simulink model "RajamaniController"  (R2018a)
settings: Solver=FixedStepDiscrete  StartTime=0.0  StopTime=inf  FixedStep=0.002  RelTol=1e-3  EnableMultiTasking=on
values from neighbouring files (symbols this model uses):
  A = [0 1 0 0; 0 A22 A23 A24; 0 0 0 1; 0 A42 A43 A44;]    [data.m]
  B1 = [0; B1_12; 0; B1_14]    [data.m]
  B2 = [0; B2_12; 0; B2_14]    [data.m]
  K = place(A, B1, P)    [data.m]
  PsiDot_des = Vx/R    (= 0.03)    [data.m]
settings Model: ExtModeTrigDuration=10000  Creator=srivats  LastModifiedBy=srivats
settings SolverCC: PositivePriorityOrder=on
settings RTWCC: SystemTargetFile=quarc_win64.tlc  TemplateMakefile=quarc_default_tmf  Description=QUARC Win64 Target
settings STFCustomTargetCC: TargetPreCompLibLocation=C:\PROGRA~3\QUARC\lib\2018a\win64\release  TargetLangStandard=C99 (ISO)  ConcurrentExecutionCompliant=on  SystemTargetFile=quarc_win64.tlc
settings GRTTargetCC: TargetPreCompLibLocation=C:\PROGRA~3\QUARC\lib\2018a\win64\release  ParMdlRefBuildCompliant=off  CompOptLevelCompliant=off  CombineOutputUpdateFcns=off  MatFileLogging=off  CPPClassGenCompliant=off  GRTInterface=on  UseToolchainInfoCompliant=off  ExtMode=on  ExtModeMexFile=quarc_comm

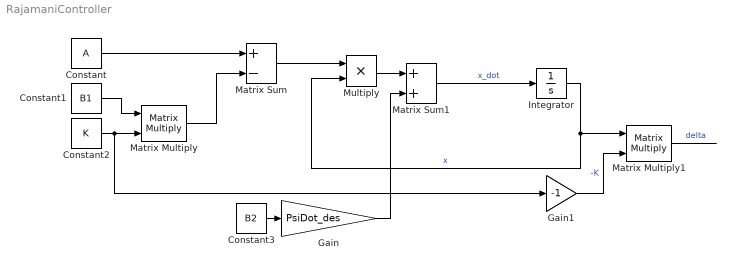
== system RajamaniController ==
  Constant : Constant  Value=A
  Constant1 : Constant  Value=B1
  Constant2 : Constant  Value=K
  Constant3 : Constant  Value=B2
  Gain : Gain  Gain=PsiDot_des
  Gain1 : Gain  Gain=-1
  Integrator : Integrator
  Matrix Sum : Sum  Inputs=+-
  Matrix Sum1 : Sum
  Matrix Multiply : Product  Multiplication=Matrix(*)
  Matrix Multiply1 : Product  Multiplication=Matrix(*)
  Multiply : Product
  wires:
  Constant/1 -> Matrix Sum/1
  Constant1/1 -> Matrix Multiply/1
  Constant2/1 -> Gain1/1, Matrix Multiply/2
  Matrix Multiply/1 -> Matrix Sum/2
  Matrix Sum/1 -> Multiply/1
  Integrator/1 -> Matrix Multiply1/1, Multiply/2  "x"
  Multiply/1 -> Matrix Sum1/1
  Gain/1 -> Matrix Sum1/2
  Constant3/1 -> Gain/1
  Matrix Sum1/1 -> Integrator/1  "x_dot"
  Gain1/1 -> Matrix Multiply1/2  "-K"
  Matrix Multiply1/1 -> ?  "delta"
